simulink model "Task_1_project"  (R2018a)
settings: Solver=VariableStepAuto  StartTime=0.0  StopTime=0.02  RelTol=1e-3
libraries: dspstat3 x2, simulink x1, dsparch4 x1, dspmathops x1
settings Model: Creator=Labiba  LastModifiedBy=Labiba

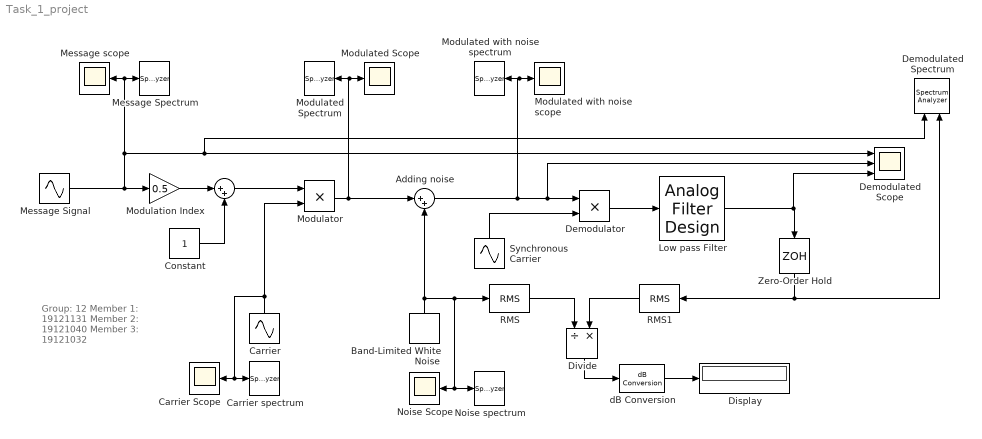
== system Task_1_project ==
  note: Group: 12
      | Member 1: 19121131
      | Member 2: 19121040
      | Member 3: 19121032
  " " : Sum  Inputs=|++
  " Adding noise" : Sum  Inputs=|++
  Band-Limited White Noise : simulink/Sources/Band-Limited White Noise  Cov=[9.000011*10^-15]  Ts=1/25000000  seed=[23341]
  Carrier : Sin  Amplitude=1.995  Frequency=2*pi*1350000  SampleTime=1/25000000
  Carrier spectrum : SpectrumAnalyzer
  Carrier Scope : Scope
  Constant : Constant
  Demodulated Scope : Scope  NumInputPorts=3
  Demodulated Spectrum : SpectrumAnalyzer  NumInputPorts=2
  Demodulator : Product
  Display : Display
  Divide : Product  Inputs=/*
  Low pass Filter : dsparch4/Analog Filter Design  method=Butterworth  filttype=Lowpass  N=8  Wlo=2*pi*1000  Whi=80  Rp=2  Rs=40
  Message scope : Scope
  Message Spectrum : SpectrumAnalyzer
  Message Signal : Sin  Frequency=2*pi*1000  SampleTime=1/25000000  VectorParams1D=off
  Modulated Scope : Scope
  Modulated Spectrum : SpectrumAnalyzer
  Modulated with noise scope : Scope
  Modulated with noise spectrum : SpectrumAnalyzer
  Modulation Index : Gain  Gain=0.5
  Modulator : Product
  Noise spectrum : SpectrumAnalyzer
  Noise Scope : Scope
  RMS : dspstat3/RMS  run=off  directionMode=Entire input  dimension=1  reset_popup=None
  RMS1 : dspstat3/RMS  run=off  directionMode=Entire input  dimension=1  reset_popup=None
  Synchronous Carrier : Sin  Amplitude=1.995  Frequency=2*pi*1350000  SampleTime=1/25000000
  Zero-Order Hold : ZeroOrderHold  SampleTime=-1
  dB Conversion : dspmathops/dB Conversion  dBtype=dB  intype=Power  R=1  fuzz=off
      settings: SourceProductName=DSP System Toolbox
  wires:
  Message Signal/1 -> Modulation Index/1, Message scope/1, Message Spectrum/1, Demodulated Spectrum/1, Demodulated Scope/1
  Synchronous Carrier/1 -> Demodulator/2
  Demodulator/1 -> Low pass Filter/1
  Low pass Filter/1 -> Zero-Order Hold/1, Demodulated Scope/3
  Carrier/1 -> Carrier Scope/1, Carrier spectrum/1, Modulator/2
  Constant/1 -> " "/2
  RMS1/1 -> Divide/2
  RMS/1 -> Divide/1
  dB Conversion/1 -> Display/1
  " Adding noise"/1 -> Demodulated Scope/2, Demodulator/1, Modulated with noise spectrum/1, Modulated with noise scope/1
  Zero-Order Hold/1 -> Demodulated Spectrum/2, RMS1/1
  Divide/1 -> dB Conversion/1
  Band-Limited White Noise/1 -> " Adding noise"/2, RMS/1, Noise spectrum/1, Noise Scope/1
  " "/1 -> Modulator/1
  Modulator/1 -> Modulated Scope/1, Modulated Spectrum/1, " Adding noise"/1
  Modulation Index/1 -> " "/1
